simulink model "Z_DCDC3_CL"  (R2024a)
settings: Solver=FixedStepDiscrete  StartTime=0.0  StopTime=Tsim_outLoop  FixedStep=Tstep  RelTol=1e-3
values from neighbouring files (symbols this model uses):
  deadtimesw = 2.8e-6    (= 2.8e-06)    [DCDC_param.m]
  ILmax = 10    [DCDC_param.m]
  Rload = VoutNom/IoutNom    (= 16.6666666667)    [DCDC_param.m]
  Tsw = 1/fsw    (= 0.0001)    [DCDC_param.m]    (also in adcpwm_setup.m)
  VinNom = 30    [DCDC_param.m]
  VoutNom = 50    [DCDC_param.m]
undefined symbols (not defined in the file or in its folder): DiscIntNeverNeededParam, kaw_i, kaw_v, ki_i, ki_v, kp_i, kp_v, Tstep, VLlim, zden_aaf, zden_plant_i, zden_plant_v, znum_aaf, znum_plant_i, znum_plant_v
libraries: simulink x10, spsTriangleGeneratorLib x6
settings Model: Creator=nicholas  LastModifiedBy=nicholas
settings RTWCC: GPUComputeCapability=3.5

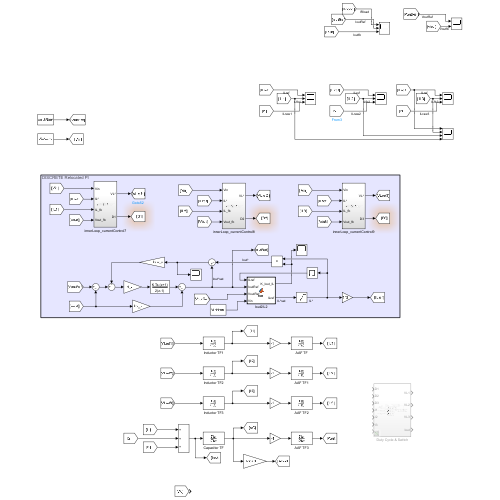
[thumbnail: Simulink's stored preview of the top-level diagram]
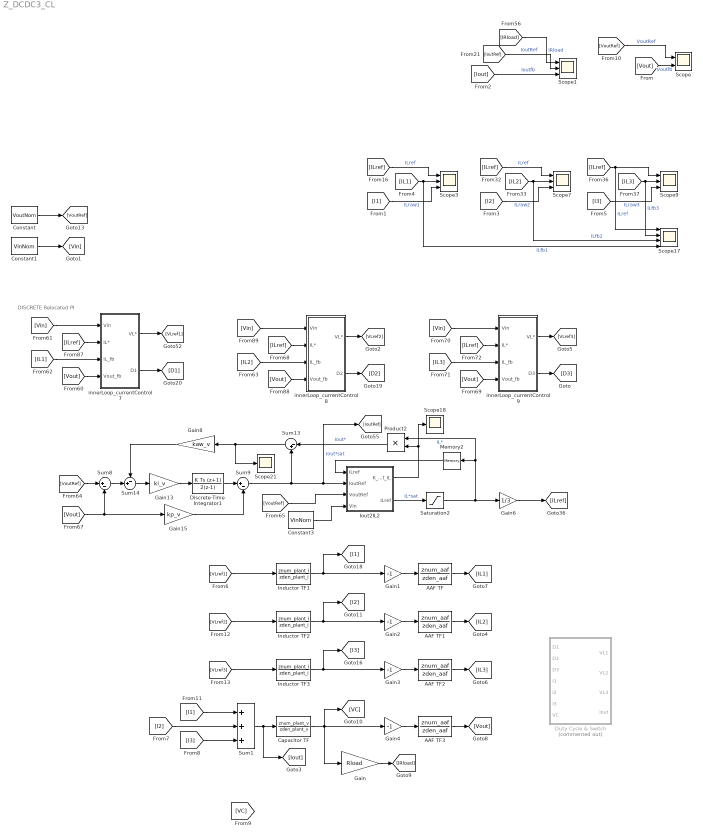
== system Z_DCDC3_CL ==
  note: DISCRETE Relocated PI
  AAF TF{,1..3} (4 alike) : DiscreteTransferFcn  Numerator=znum_aaf  Denominator=zden_aaf
  Capacitor TF : DiscreteTransferFcn  Numerator=znum_plant_v  Denominator=zden_plant_v
  Constant : Constant  Value=VoutNom
  Constant1 : Constant  Value=VinNom
  Constant3 : Constant  Value=VinNom
  Discrete-Time Integrator1 : DiscreteIntegrator  IntegratorMethod=Integration: Trapezoidal  SampleTime=Tsw  ICPrevOutput=DiscIntNeverNeededParam  ICPrevScaledInput=DiscIntNeverNeededParam
  Duty Cycle & Switch : Subsystem  Commented=on
  Gain : Gain  Gain=Rload
  Gain{1..4} (4 alike) : Gain  Gain=-1
  Gain13 : Gain  Gain=ki_v
  Gain15 : Gain  Gain=kp_v
  Gain6 : Gain  Gain=1/3
  Gain8 : Gain  Gain=kaw_v
  Inductor TF1 : DiscreteTransferFcn  Numerator=znum_plant_i  Denominator=zden_plant_i
  Inductor TF2 : DiscreteTransferFcn  Numerator=znum_plant_i  Denominator=zden_plant_i
  Inductor TF3 : DiscreteTransferFcn  Numerator=znum_plant_i  Denominator=zden_plant_i
  Iout2IL2 : MATLAB Function  TreatAsAtomicUnit=on
  Memory2 : Memory
  Product2 : Product
  Saturation2 : Saturate  UpperLimit=ILmax  LowerLimit=-ILmax
  Scope : Scope  NumInputPorts=2
  Scope{1,3,7,9} (4 alike) : Scope  NumInputPorts=3
  Scope17 : Scope  NumInputPorts=4
  Scope18 : Scope
  Scope21 : Scope
  Sum1 : Sum  Inputs=+++
  Sum13 : Sum  Inputs=|-+
  Sum14 : Sum  Inputs=-+|
  Sum8 : Sum  Inputs=|+-
  Sum9 : Sum  Inputs=|+-
  innerLoop_currentControl7 : Subsystem
  innerLoop_currentControl8 : Subsystem
  innerLoop_currentControl9 : Subsystem
  wires:
  [Iout] -> Scope1/3  "Ioutfb"
  [Vout] -> Scope/2  "Voutfb"
  [IL1] -> Scope17/4, Scope3/2  "ILfb1"
  [ILref] -> Scope3/1  "ILref"
  [VoutRef] -> Scope/1  "VoutRef"
  [IoutRef] -> Scope1/2  "IoutRef"
  Constant/1 -> [VoutRef]
  [IL2] -> Scope7/2, Scope17/3  "ILfb2"
  [ILref] -> Scope7/1  "ILref"
  [IL3] -> Scope17/2, Scope9/2  "ILfb3"
  [ILref] -> Scope17/1, Scope9/1  "ILref"
  [IRload] -> Scope1/1  "IRload"
  [I1] -> Scope3/3  "ILraw1"
  [I2] -> Scope7/3  "ILraw2"
  [I3] -> Scope9/3  "ILraw3"
  Saturation2/1 -> Product2/1, Memory2/1, Gain6/1  "IL*"
  [IL1] -> innerLoop_currentControl7/3(IL_fb)
  [Vout] -> innerLoop_currentControl8/4(Vout_fb)
  [Vin] -> innerLoop_currentControl9/1(Vin)
  Gain13/1 -> Discrete-Time Integrator1/1
  [VoutRef] -> Sum8/1
  [Vout] -> innerLoop_currentControl7/4(Vout_fb)
  [Vin] -> innerLoop_currentControl7/1(Vin)
  Discrete-Time Integrator1/1 -> Sum9/1
  Constant3/1 -> Iout2IL2/4(Vin)
  [ILref] -> innerLoop_currentControl8/2(IL*)
  Product2/1 -> Sum13/1  "Iout*"
  Iout2IL2/2(ILref) -> Saturation2/1  "IL*sat"
  [IL3] -> innerLoop_currentControl9/3(IL_fb)
  Iout2IL2/1(K_Iout_IL) -> Product2/2, Scope18/1
  [IL2] -> innerLoop_currentControl8/3(IL_fb)
  [VoutRef] -> Iout2IL2/3(VoutRef)
  Memory2/1 -> Iout2IL2/1("ILref ")
  Gain8/1 -> Sum14/1
  Gain6/1 -> [ILref]
  [Vout] -> Gain15/1, Sum8/2
  Sum9/1 -> Sum13/2, Iout2IL2/2(IoutRef), [IoutRef]  "Iout*sat"
  [ILref] -> innerLoop_currentControl7/2(IL*)
  Sum8/1 -> Sum14/2
  Sum14/1 -> Gain13/1
  [Vin] -> innerLoop_currentControl8/1(Vin)
  [ILref] -> innerLoop_currentControl9/2(IL*)
  [Vout] -> innerLoop_currentControl9/4(Vout_fb)
  Sum13/1 -> Scope21/1, Gain8/1
  Gain15/1 -> Sum9/2
  Sum1/1 -> [Iout], Capacitor TF/1
  Inductor TF1/1 -> [I1], Gain1/1
  Inductor TF2/1 -> [I2], Gain2/1
  Inductor TF3/1 -> [I3], Gain3/1
  Capacitor TF/1 -> Gain/1, [VC], Gain4/1
  AAF TF3/1 -> [Vout]
  AAF TF2/1 -> [IL3]
  AAF TF1/1 -> [IL2]
  AAF TF/1 -> [IL1]
  Gain/1 -> [IRload]
  innerLoop_currentControl9/2(D3) -> [D3]
  innerLoop_currentControl8/2(D2) -> [D2]
  innerLoop_currentControl7/2(D1) -> [D1]
  Constant1/1 -> [Vin]
  Gain1/1 -> AAF TF/1
  Gain2/1 -> AAF TF1/1
  Gain3/1 -> AAF TF2/1
  Gain4/1 -> AAF TF3/1
  [I1] -> Sum1/1
  [I2] -> Sum1/2
  [I3] -> Sum1/3
  [VLref1] -> Inductor TF1/1
  innerLoop_currentControl7/1(VL*) -> [VLref1]
  innerLoop_currentControl8/1(VL*) -> [VLref2]
  innerLoop_currentControl9/1(VL*) -> [VLref3]
  [VLref2] -> Inductor TF2/1
  [VLref3] -> Inductor TF3/1

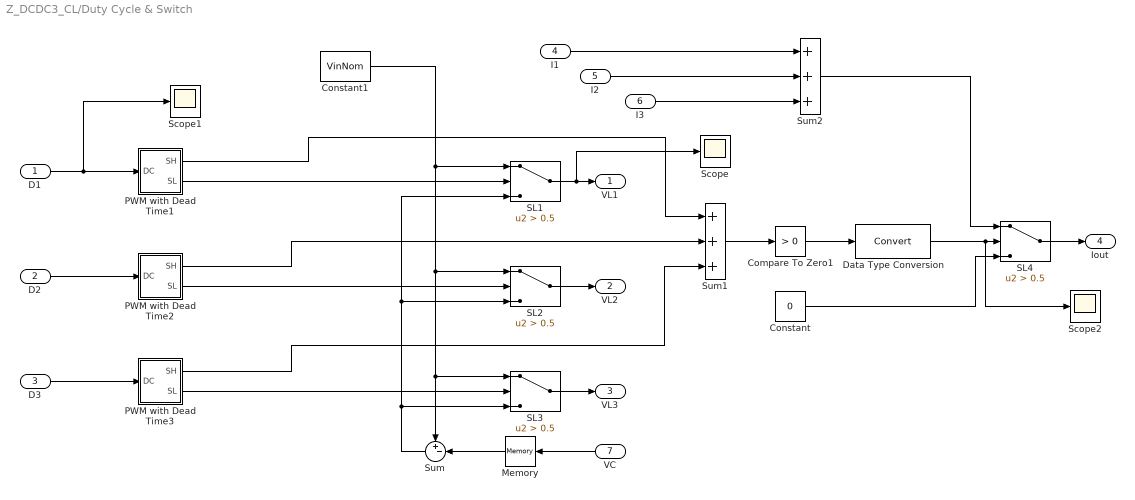
== system Z_DCDC3_CL/Duty Cycle & Switch ==
  D1 : Inport
  D2 : Inport  Port=2
  D3 : Inport  Port=3
  I1 : Inport  Port=4
  I2 : Inport  Port=5
  I3 : Inport  Port=6
  VC : Inport  Port=7
  Compare To Zero1 : simulink/Logic and Bit Operations/Compare To Zero  relop=>  OutDataTypeStr=boolean
  Constant : Constant  Value=0
  Constant1 : Constant  Value=VinNom
  Data Type Conversion : DataTypeConversion  SaturateOnIntegerOverflow=off  RndMeth=Floor
  Memory : Memory
  PWM with Dead Time1 : Subsystem
  PWM with Dead Time2 : Subsystem
  PWM with Dead Time3 : Subsystem
  SL{1..4} (4 alike) : Switch  Criteria=u2 > Threshold  Threshold=0.5  SaturateOnIntegerOverflow=off  InputSameDT=off
  Scope : Scope
  Scope1 : Scope
  Scope2 : Scope
  Sum : Sum  Inputs=+-|
  Sum1 : Sum  Inputs=+++
  Sum2 : Sum  Inputs=+++
  VL1 : Outport
  VL2 : Outport  Port=2
  VL3 : Outport  Port=3
  Iout : Outport  Port=4
  wires:
  D1/1 -> Scope1/1, PWM with Dead Time1/1(DC)
  D2/1 -> PWM with Dead Time2/1(DC)
  PWM with Dead Time2/2(SL) -> SL2/2
  PWM with Dead Time3/2(SL) -> SL3/2
  Constant1/1 -> SL1/1, SL2/1, SL3/1, Sum/1
  PWM with Dead Time1/2(SL) -> SL1/2
  PWM with Dead Time3/1(SH) -> Sum1/3
  PWM with Dead Time2/1(SH) -> Sum1/2
  PWM with Dead Time1/1(SH) -> Sum1/1
  SL1/1 -> Scope/1, VL1/1
  SL2/1 -> VL2/1
  SL3/1 -> VL3/1
  Sum/1 -> SL1/3, SL2/3, SL3/3
  Sum1/1 -> Compare To Zero1/1
  Compare To Zero1/1 -> Data Type Conversion/1
  Sum2/1 -> SL4/1
  Constant/1 -> SL4/3
  SL4/1 -> Iout/1
  I1/1 -> Sum2/1
  I2/1 -> Sum2/2
  I3/1 -> Sum2/3
  Data Type Conversion/1 -> Scope2/1, SL4/2
  D3/1 -> PWM with Dead Time3/1(DC)
  VC/1 -> Memory/1
  Memory/1 -> Sum/2

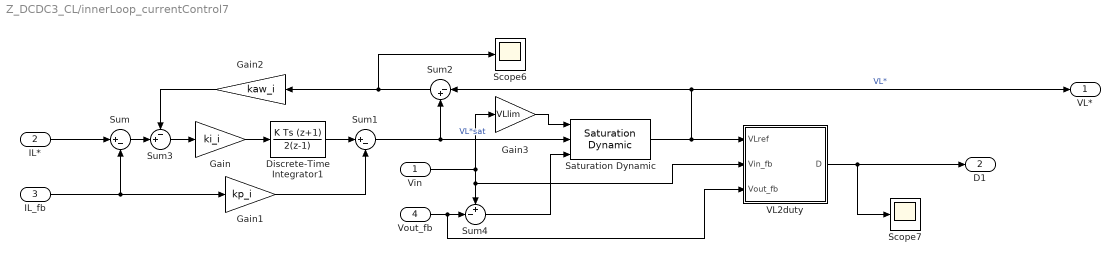
== system Z_DCDC3_CL/innerLoop_currentControl7 ==
  Vin : Inport
  IL* : Inport  Port=2
  IL_fb : Inport  Port=3
  Vout_fb : Inport  Port=4
  Discrete-Time Integrator1 : DiscreteIntegrator  IntegratorMethod=Integration: Trapezoidal  SampleTime=Tsw  ICPrevOutput=DiscIntNeverNeededParam  ICPrevScaledInput=DiscIntNeverNeededParam
  Gain : Gain  Gain=ki_i
  Gain1 : Gain  Gain=kp_i
  Gain2 : Gain  Gain=kaw_i
  Gain3 : Gain  Gain=VLlim
  Saturation Dynamic : simulink/Discontinuities/Saturation Dynamic  OutMin=[]  OutMax=[]  OutDataTypeStr=Inherit: Same as second input  OutDataType=fixdt(1, 16)  OutScaling=2^-10  DoSatur=off
  Scope6 : Scope
  Scope7 : Scope
  Sum : Sum  Inputs=|+-
  Sum1 : Sum  Inputs=|+-
  Sum2 : Sum  Inputs=|-+
  Sum3 : Sum  Inputs=-+|
  Sum4 : Sum  Inputs=+-|
  VL2duty : MATLAB Function  TreatAsAtomicUnit=on
  VL* : Outport
  D1 : Outport  Port=2
  wires:
  VL2duty/1(D) -> D1/1, Scope7/1
  Sum/1 -> Sum3/2
  Gain3/1 -> Saturation Dynamic/1
  Gain1/1 -> Sum1/2
  Sum3/1 -> Gain/1
  Gain/1 -> Discrete-Time Integrator1/1
  Gain2/1 -> Sum3/1
  Vin/1 -> VL2duty/2(Vin_fb), Sum4/1, Gain3/1
  Sum1/1 -> Saturation Dynamic/2, Sum2/2  "VL*sat"
  Sum4/1 -> Saturation Dynamic/3
  Sum2/1 -> Gain2/1, Scope6/1
  Saturation Dynamic/1 -> VL2duty/1(VLref), VL*/1, Sum2/1  "VL*"
  IL_fb/1 -> Sum/2, Gain1/1
  Vout_fb/1 -> VL2duty/3(Vout_fb), Sum4/2
  Discrete-Time Integrator1/1 -> Sum1/1
  IL*/1 -> Sum/1

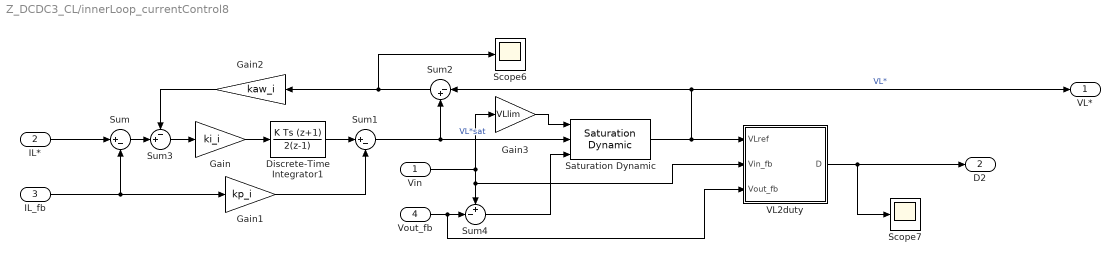
== system Z_DCDC3_CL/innerLoop_currentControl8 ==
  Vin : Inport
  IL* : Inport  Port=2
  IL_fb : Inport  Port=3
  Vout_fb : Inport  Port=4
  Discrete-Time Integrator1 : DiscreteIntegrator  IntegratorMethod=Integration: Trapezoidal  SampleTime=Tsw  ICPrevOutput=DiscIntNeverNeededParam  ICPrevScaledInput=DiscIntNeverNeededParam
  Gain : Gain  Gain=ki_i
  Gain1 : Gain  Gain=kp_i
  Gain2 : Gain  Gain=kaw_i
  Gain3 : Gain  Gain=VLlim
  Saturation Dynamic : simulink/Discontinuities/Saturation Dynamic  OutMin=[]  OutMax=[]  OutDataTypeStr=Inherit: Same as second input  OutDataType=fixdt(1, 16)  OutScaling=2^-10  DoSatur=off
  Scope6 : Scope
  Scope7 : Scope
  Sum : Sum  Inputs=|+-
  Sum1 : Sum  Inputs=|+-
  Sum2 : Sum  Inputs=|-+
  Sum3 : Sum  Inputs=-+|
  Sum4 : Sum  Inputs=+-|
  VL2duty : MATLAB Function  TreatAsAtomicUnit=on
  VL* : Outport
  D2 : Outport  Port=2
  wires:
  Sum/1 -> Sum3/2
  Gain3/1 -> Saturation Dynamic/1
  Gain1/1 -> Sum1/2
  Sum3/1 -> Gain/1
  Gain/1 -> Discrete-Time Integrator1/1
  Gain2/1 -> Sum3/1
  Vin/1 -> VL2duty/2(Vin_fb), Sum4/1, Gain3/1
  Sum1/1 -> Saturation Dynamic/2, Sum2/2  "VL*sat"
  Sum4/1 -> Saturation Dynamic/3
  Sum2/1 -> Gain2/1, Scope6/1
  Saturation Dynamic/1 -> VL2duty/1(VLref), VL*/1, Sum2/1  "VL*"
  Vout_fb/1 -> VL2duty/3(Vout_fb), Sum4/2
  Discrete-Time Integrator1/1 -> Sum1/1
  IL*/1 -> Sum/1
  VL2duty/1(D) -> D2/1, Scope7/1
  IL_fb/1 -> Sum/2, Gain1/1

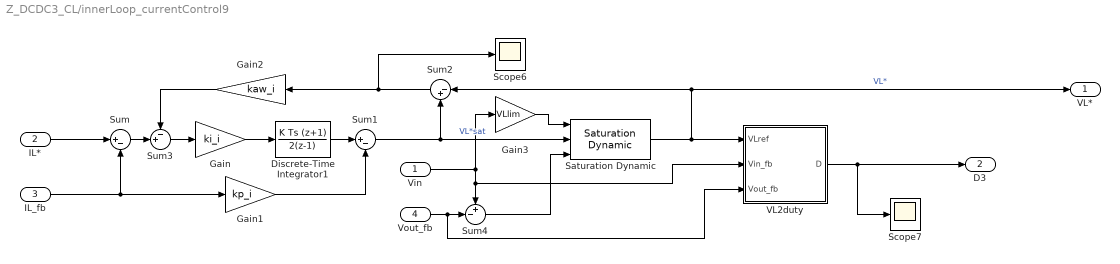
== system Z_DCDC3_CL/innerLoop_currentControl9 ==
  Vin : Inport
  IL* : Inport  Port=2
  IL_fb : Inport  Port=3
  Vout_fb : Inport  Port=4
  Discrete-Time Integrator1 : DiscreteIntegrator  IntegratorMethod=Integration: Trapezoidal  SampleTime=Tsw  ICPrevOutput=DiscIntNeverNeededParam  ICPrevScaledInput=DiscIntNeverNeededParam
  Gain : Gain  Gain=ki_i
  Gain1 : Gain  Gain=kp_i
  Gain2 : Gain  Gain=kaw_i
  Gain3 : Gain  Gain=VLlim
  Saturation Dynamic : simulink/Discontinuities/Saturation Dynamic  OutMin=[]  OutMax=[]  OutDataTypeStr=Inherit: Same as second input  OutDataType=fixdt(1, 16)  OutScaling=2^-10  DoSatur=off
  Scope6 : Scope
  Scope7 : Scope
  Sum : Sum  Inputs=|+-
  Sum1 : Sum  Inputs=|+-
  Sum2 : Sum  Inputs=|-+
  Sum3 : Sum  Inputs=-+|
  Sum4 : Sum  Inputs=+-|
  VL2duty : MATLAB Function  TreatAsAtomicUnit=on
  VL* : Outport
  D3 : Outport  Port=2
  wires:
  Sum/1 -> Sum3/2
  Gain3/1 -> Saturation Dynamic/1
  Gain1/1 -> Sum1/2
  Sum3/1 -> Gain/1
  Gain/1 -> Discrete-Time Integrator1/1
  Gain2/1 -> Sum3/1
  Vin/1 -> VL2duty/2(Vin_fb), Sum4/1, Gain3/1
  Sum1/1 -> Saturation Dynamic/2, Sum2/2  "VL*sat"
  Sum4/1 -> Saturation Dynamic/3
  Sum2/1 -> Gain2/1, Scope6/1
  Saturation Dynamic/1 -> VL2duty/1(VLref), VL*/1, Sum2/1  "VL*"
  IL_fb/1 -> Sum/2, Gain1/1
  Vout_fb/1 -> VL2duty/3(Vout_fb), Sum4/2
  Discrete-Time Integrator1/1 -> Sum1/1
  IL*/1 -> Sum/1
  VL2duty/1(D) -> D3/1, Scope7/1

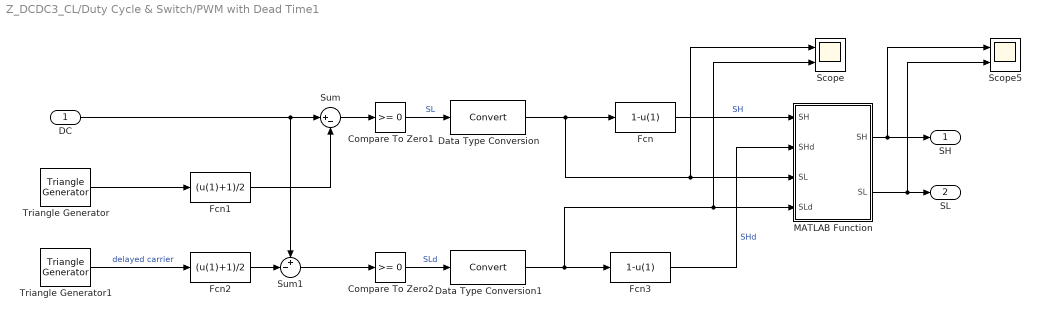
== system Z_DCDC3_CL/Duty Cycle & Switch/PWM with Dead Time1 ==
  DC : Inport
  Compare To Zero1 : simulink/Logic and Bit Operations/Compare To Zero  relop=>=  OutDataTypeStr=boolean
  Compare To Zero2 : simulink/Logic and Bit Operations/Compare To Zero  relop=>=  OutDataTypeStr=boolean
  Data Type Conversion : DataTypeConversion  SaturateOnIntegerOverflow=off  RndMeth=Floor
  Data Type Conversion1 : DataTypeConversion  SaturateOnIntegerOverflow=off  RndMeth=Floor
  Fcn : Fcn  Expr=1-u(1)
  Fcn1 : Fcn  Expr=(u(1)+1)/2
  Fcn2 : Fcn  Expr=(u(1)+1)/2
  Fcn3 : Fcn  Expr=1-u(1)
  MATLAB Function : MATLAB Function  TreatAsAtomicUnit=on
  Scope : Scope  NumInputPorts=2
  Scope5 : Scope  NumInputPorts=2
  Sum : Sum  Inputs=|+-
  Sum1 : Sum  Inputs=+-|
  Triangle Generator : spsTriangleGeneratorLib/Triangle Generator  Freq=fsw  Phase=0  Ts=Tstep
  Triangle Generator1 : spsTriangleGeneratorLib/Triangle Generator  Freq=fsw  Phase=-(deadtimesw/Tsw)*360  Ts=Tstep
  SH : Outport
  SL : Outport  Port=2
  wires:
  Compare To Zero1/1 -> Data Type Conversion/1  "SL"
  Fcn/1 -> MATLAB Function/1("SH ")  "SH"
  MATLAB Function/2(SL) -> SL/1, Scope5/2
  MATLAB Function/1(SH) -> SH/1, Scope5/1
  DC/1 -> Sum1/1, Sum/1
  Triangle Generator/1 -> Fcn1/1
  Sum/1 -> Compare To Zero1/1
  Fcn1/1 -> Sum/2
  Triangle Generator1/1 -> Fcn2/1  "delayed carrier"
  Sum1/1 -> Compare To Zero2/1
  Fcn2/1 -> Sum1/2
  Compare To Zero2/1 -> Data Type Conversion1/1  "SLd"
  Fcn3/1 -> MATLAB Function/2(SHd)  "SHd"
  Data Type Conversion/1 -> Fcn/1, Scope/1, MATLAB Function/3("SL ")
  Data Type Conversion1/1 -> Fcn3/1, Scope/2, MATLAB Function/4(SLd)

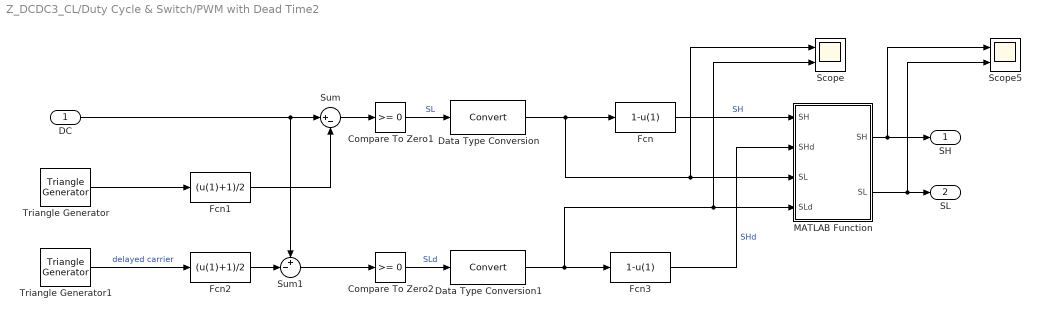
== system Z_DCDC3_CL/Duty Cycle & Switch/PWM with Dead Time2 ==
  DC : Inport
  Compare To Zero1 : simulink/Logic and Bit Operations/Compare To Zero  relop=>=  OutDataTypeStr=boolean
  Compare To Zero2 : simulink/Logic and Bit Operations/Compare To Zero  relop=>=  OutDataTypeStr=boolean
  Data Type Conversion : DataTypeConversion  SaturateOnIntegerOverflow=off  RndMeth=Floor
  Data Type Conversion1 : DataTypeConversion  SaturateOnIntegerOverflow=off  RndMeth=Floor
  Fcn : Fcn  Expr=1-u(1)
  Fcn1 : Fcn  Expr=(u(1)+1)/2
  Fcn2 : Fcn  Expr=(u(1)+1)/2
  Fcn3 : Fcn  Expr=1-u(1)
  MATLAB Function : MATLAB Function  TreatAsAtomicUnit=on
  Scope : Scope  NumInputPorts=2
  Scope5 : Scope  NumInputPorts=2
  Sum : Sum  Inputs=|+-
  Sum1 : Sum  Inputs=+-|
  Triangle Generator : spsTriangleGeneratorLib/Triangle Generator  Freq=fsw  Phase=120  Ts=Tstep
  Triangle Generator1 : spsTriangleGeneratorLib/Triangle Generator  Freq=fsw  Phase=120-(deadtimesw/Tsw)*360  Ts=Tstep
  SH : Outport
  SL : Outport  Port=2
  wires:
  Compare To Zero1/1 -> Data Type Conversion/1  "SL"
  Fcn/1 -> MATLAB Function/1("SH ")  "SH"
  MATLAB Function/2(SL) -> SL/1, Scope5/2
  MATLAB Function/1(SH) -> SH/1, Scope5/1
  DC/1 -> Sum1/1, Sum/1
  Triangle Generator/1 -> Fcn1/1
  Sum/1 -> Compare To Zero1/1
  Fcn1/1 -> Sum/2
  Triangle Generator1/1 -> Fcn2/1  "delayed carrier"
  Sum1/1 -> Compare To Zero2/1
  Fcn2/1 -> Sum1/2
  Compare To Zero2/1 -> Data Type Conversion1/1  "SLd"
  Fcn3/1 -> MATLAB Function/2(SHd)  "SHd"
  Data Type Conversion/1 -> Fcn/1, Scope/1, MATLAB Function/3("SL ")
  Data Type Conversion1/1 -> Fcn3/1, Scope/2, MATLAB Function/4(SLd)

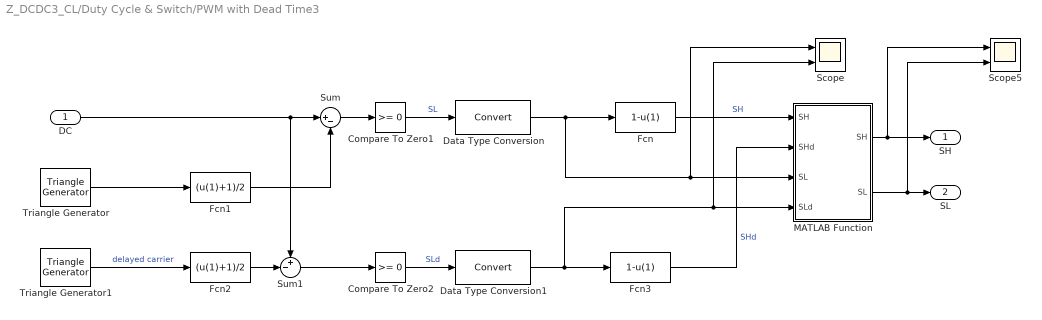
== system Z_DCDC3_CL/Duty Cycle & Switch/PWM with Dead Time3 ==
  DC : Inport
  Compare To Zero1 : simulink/Logic and Bit Operations/Compare To Zero  relop=>=  OutDataTypeStr=boolean
  Compare To Zero2 : simulink/Logic and Bit Operations/Compare To Zero  relop=>=  OutDataTypeStr=boolean
  Data Type Conversion : DataTypeConversion  SaturateOnIntegerOverflow=off  RndMeth=Floor
  Data Type Conversion1 : DataTypeConversion  SaturateOnIntegerOverflow=off  RndMeth=Floor
  Fcn : Fcn  Expr=1-u(1)
  Fcn1 : Fcn  Expr=(u(1)+1)/2
  Fcn2 : Fcn  Expr=(u(1)+1)/2
  Fcn3 : Fcn  Expr=1-u(1)
  MATLAB Function : MATLAB Function  TreatAsAtomicUnit=on
  Scope : Scope  NumInputPorts=2
  Scope5 : Scope  NumInputPorts=2
  Sum : Sum  Inputs=|+-
  Sum1 : Sum  Inputs=+-|
  Triangle Generator : spsTriangleGeneratorLib/Triangle Generator  Freq=fsw  Phase=240  Ts=Tstep
  Triangle Generator1 : spsTriangleGeneratorLib/Triangle Generator  Freq=fsw  Phase=240-(deadtimesw/Tsw)*360  Ts=Tstep
  SH : Outport
  SL : Outport  Port=2
  wires:
  Compare To Zero1/1 -> Data Type Conversion/1  "SL"
  Fcn/1 -> MATLAB Function/1("SH ")  "SH"
  MATLAB Function/2(SL) -> SL/1, Scope5/2
  MATLAB Function/1(SH) -> SH/1, Scope5/1
  DC/1 -> Sum1/1, Sum/1
  Triangle Generator/1 -> Fcn1/1
  Sum/1 -> Compare To Zero1/1
  Fcn1/1 -> Sum/2
  Triangle Generator1/1 -> Fcn2/1  "delayed carrier"
  Sum1/1 -> Compare To Zero2/1
  Fcn2/1 -> Sum1/2
  Compare To Zero2/1 -> Data Type Conversion1/1  "SLd"
  Fcn3/1 -> MATLAB Function/2(SHd)  "SHd"
  Data Type Conversion/1 -> Fcn/1, Scope/1, MATLAB Function/3("SL ")
  Data Type Conversion1/1 -> Fcn3/1, Scope/2, MATLAB Function/4(SLd)

== matlab function Z_DCDC3_CL/Duty Cycle & Switch/PWM with Dead Time1/MATLAB Function ==
  data: SH input; SHd input; SH output; SL output; SL input; SLd input
function [SH,SL] = fcn(SH,SHd,SL,SLd)

if SHd + SH > 1
    SH = 1;
else
    SH = 0;
end

if SLd + SL > 1
    SL = 1;
else
    SL = 0;
end

== matlab function Z_DCDC3_CL/Duty Cycle & Switch/PWM with Dead Time2/MATLAB Function ==
  data: SH input; SHd input; SH output; SL output; SL input; SLd input
function [SH,SL] = fcn(SH,SHd,SL,SLd)

if SHd + SH > 1
    SH = 1;
else
    SH = 0;
end

if SLd + SL > 1
    SL = 1;
else
    SL = 0;
end

== matlab function Z_DCDC3_CL/Duty Cycle & Switch/PWM with Dead Time3/MATLAB Function ==
  data: SH input; SHd input; SH output; SL output; SL input; SLd input
function [SH,SL] = fcn(SH,SHd,SL,SLd)

if SHd + SH > 1
    SH = 1;
else
    SH = 0;
end

if SLd + SL > 1
    SL = 1;
else
    SL = 0;
end

== matlab function Z_DCDC3_CL/Iout2IL2 ==
  data: K_Iout_IL output; ILref input; IoutRef input; VoutRef input; Vin input; ILref output; RserL parameter
function [K_Iout_IL,ILref] = fcn(ILref,IoutRef,VoutRef,Vin,RserL)

if VoutRef < Vin
    VoutRef = Vin;
end
K_Iout_IL = (Vin - RserL*ILref) / VoutRef;
ILref = IoutRef / K_Iout_IL;

== matlab function Z_DCDC3_CL/innerLoop_currentControl7/VL2duty ==
  data: VLref input; D output; Vin_fb input; Vout_fb input
function D = fcn(VLref,Vin_fb,Vout_fb)

D = min([1 max([0 1 + (VLref - Vin_fb)/Vout_fb])]);

== matlab function Z_DCDC3_CL/innerLoop_currentControl8/VL2duty ==
  data: VLref input; D output; Vin_fb input; Vout_fb input
function D = fcn(VLref,Vin_fb,Vout_fb)

D = min([1 max([0 1 + (VLref - Vin_fb)/Vout_fb])]);

== matlab function Z_DCDC3_CL/innerLoop_currentControl9/VL2duty ==
  data: VLref input; D output; Vin_fb input; Vout_fb input
function D = fcn(VLref,Vin_fb,Vout_fb)

D = min([1 max([0 1 + (VLref - Vin_fb)/Vout_fb])]);
